simulink library "LU_TEG"  (R2015a)
settings: Solver=ode45  StartTime=0.0  StopTime=10.0  RelTol=1e-3
undefined symbols (not defined in the file): a, a_hxr, B, b_hxr, C_ap, C_cxr, C_hxr, ca1, ca2, ca3, cb1, cb2, cb3, ct1, ct2, Di_cxr, f, k_gap, l, l_cw, l_hxr, l_TEM, M, M_ap, M_cxr, M_hxr, n, N, Nf_hxr, P, plate_fin_hxr_A, side, T1, T1_T2, T_cint, T_hint, tf_hxr, Tune_er, Tune_tr
(part 2 of 2)

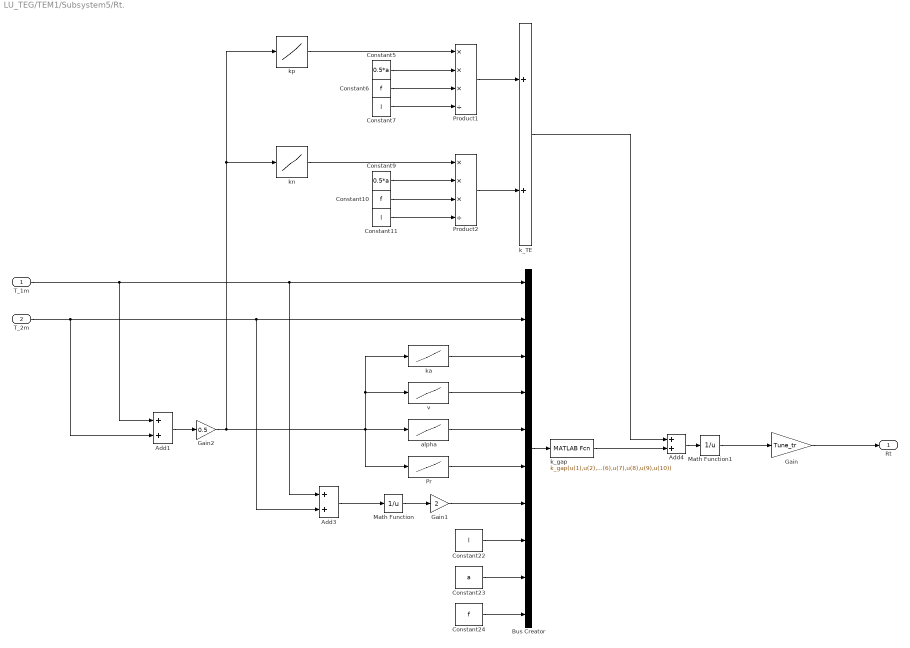
== system LU_TEG/TEM1/Subsystem5/Rt. ==
  T_1m : Inport
  T_2m : Inport  Port=2
  Add1 : Sum
  Add3 : Sum
  Add4 : Sum
  Bus Creator : BusCreator  Inputs=10
  Constant10 : Constant  Value=f
  Constant11 : Constant  Value=l
  Constant22 : Constant  Value=l
  Constant23 : Constant  Value=a
  Constant24 : Constant  Value=f
  Constant5 : Constant  Value=0.5*a
  Constant6 : Constant  Value=f
  Constant7 : Constant  Value=l
  Constant9 : Constant  Value=0.5*a
  Gain : Gain  Gain=Tune_tr
  Gain1 : Gain  Gain=2
  Gain2 : Gain  Gain=0.5
  Math Function : Math  Operator=reciprocal  SaturateOnIntegerOverflow=on
  Math Function1 : Math  Operator=reciprocal  SaturateOnIntegerOverflow=on
  Pr : Lookup_n-D  NumberOfTableDimensions=1  BreakpointsForDimension1=|  Table=|  InterpMethod=Cubic spline  ExtrapMethod=Cubic spline  RndMeth=Simplest  InputSameDT=on
      BreakpointsForDimension1=|
      | [293
      | 313
      | 333
      | 353
      | 373
      | 393
      | 413
      | 433
      | 453
      | 473
      | 493
      | 513
      | 533
      | 553
      | 573
      | 593
      | 613
      | 633
      | 653
      | 673
      | 693
      | 713
      | 733
      | 753
      | 773
      | 793
      | 813
      | 833
      | 853
      | 873
      | 900
      | 920
      | 940
      | 960
      | 980
      | 1000
      | 1020
      | 1040
      | 1060
      | 1080
      | 1100
      | 1120
      | 1140
      | 1160
      | 1180
      | 1200
      | 1220
      | 1240
      | 1260
      | 1280
      | 1300
      | 1320
      | 1340
      | 1360
      | 1380
      | 1400
      | 1420
      | 1440
      | 1460
      | 1480]
      Table=|
      | [0.70868
      | 0.70388
      | 0.69972
      | 0.6964
      | 0.6924
      | 0.68912
      | 0.68696
      | 0.68536
      | 0.68376
      | 0.68216
      | 0.68056
      | 0.68
      | 0.68
      | 0.68
      | 0.68
      | 0.68
      | 0.68052
      | 0.68132
      | 0.68212
      | 0.68292
      | 0.68372
      | 0.68478
      | 0.68598
      | 0.68718
      | 0.68838
      | 0.68958
      | 0.69078
      | 0.69198
      | 0.69318
      | 0.69438
      | 0.696
      | 0.6972
      | 0.6984
      | 0.6996
      | 0.7008
      | 0.702
      | 0.7028
      | 0.7036
      | 0.7046
      | 0.7058
      | 0.707
      | 0.7078
      | 0.7086
      | 0.7094
      | 0.7102
      | 0.711
      | 0.7118
      | 0.7126
      | 0.7134
      | 0.7142
      | 0.715
      | 0.7158
      | 0.7166
      | 0.7174
      | 0.7182
      | 0.719
      | 0.7196
      | 0.7202
      | 0.7208
      | 0.7214
      | ]
  Product1 : Product  Inputs=***/
  Product2 : Product  Inputs=***/
  alpha : Lookup_n-D  NumberOfTableDimensions=1  BreakpointsForDimension1=|  Table=|  InterpMethod=Cubic spline  ExtrapMethod=Cubic spline  RndMeth=Simplest  InputSameDT=on
      BreakpointsForDimension1=|
      | [293
      | 313
      | 333
      | 353
      | 373
      | 393
      | 413
      | 433
      | 453
      | 473
      | 493
      | 513
      | 533
      | 553
      | 573
      | 593
      | 613
      | 633
      | 653
      | 673
      | 693
      | 713
      | 733
      | 753
      | 773
      | 793
      | 813
      | 833
      | 853
      | 873
      | 900
      | 920
      | 940
      | 960
      | 980
      | 1000
      | 1020
      | 1040
      | 1060
      | 1080
      | 1100
      | 1120
      | 1140
      | 1160
      | 1180
      | 1200
      | 1220
      | 1240
      | 1260
      | 1280
      | 1300
      | 1320
      | 1340
      | 1360
      | 1380
      | 1400
      | 1420
      | 1440
      | 1460
      | 1480]
      Table=|
      | [2.14551E-05
      | 2.42197E-05
      | 2.71451E-05
      | 3.01755E-05
      | 3.32992E-05
      | 3.65423E-05
      | 3.98418E-05
      | 4.32631E-05
      | 4.67259E-05
      | 5.03421E-05
      | 5.40342E-05
      | 5.77836E-05
      | 6.16602E-05
      | 6.5511E-05
      | 6.94474E-05
      | 7.35134E-05
      | 7.75786E-05
      | 8.18073E-05
      | 8.60163E-05
      | 9.03078E-05
      | 9.47366E-05
      | 9.91488E-05
      | 0.000103728
      | 0.000108175
      | 0.000112784
      | 0.000117529
      | 0.000122257
      | 0.000127153
      | 0.000132003
      | 0.000137003
      | 0.000142748
      | 0.000147552
      | 0.000152555
      | 0.00015755
      | 0.00016252
      | 0.000167688
      | 0.000172675
      | 0.000178002
      | 0.000183174
      | 0.000188489
      | 0.00019383
      | 0.000199144
      | 0.000204639
      | 0.000210134
      | 0.000215613
      | 0.000221274
      | 0.000226733
      | 0.000232362
      | 0.000238009
      | 0.000243871
      | 0.000249704
      | 0.000255298
      | 0.000261271
      | 0.000267061
      | 0.000273104
      | 0.00027932
      | 0.000285171
      | 0.000290933
      | 0.000297092
      | 0.000303417
      | ]
  k_TE : Sum
  k_gap : MATLABFcn  MATLABFcn=k_gap(u(1),u(2),u(3),u(4),u(5),u(6),u(7),u(8),u(9),u(10))
  ka : Lookup_n-D  NumberOfTableDimensions=1  BreakpointsForDimension1=|  Table=|  InterpMethod=Cubic spline  ExtrapMethod=Cubic spline  RndMeth=Simplest  InputSameDT=on
      BreakpointsForDimension1=|
      | [293
      | 313
      | 333
      | 353
      | 373
      | 393
      | 413
      | 433
      | 453
      | 473
      | 493
      | 513
      | 533
      | 553
      | 573
      | 593
      | 613
      | 633
      | 653
      | 673
      | 693
      | 713
      | 733
      | 753
      | 773
      | 793
      | 813
      | 833
      | 853
      | 873
      | 900
      | 920
      | 940
      | 960
      | 980
      | 1000
      | 1020
      | 1040
      | 1060
      | 1080
      | 1100
      | 1120
      | 1140
      | 1160
      | 1180
      | 1200
      | 1220
      | 1240
      | 1260
      | 1280
      | 1300
      | 1320
      | 1340
      | 1360
      | 1380
      | 1400
      | 1420
      | 1440
      | 1460
      | 1480]
      Table=|
      | [0.02568
      | 0.02716
      | 0.02861
      | 0.03003
      | 0.03142
      | 0.03279
      | 0.03412
      | 0.03544
      | 0.03673
      | 0.03801
      | 0.03926
      | 0.0405
      | 0.04172
      | 0.04293
      | 0.04413
      | 0.04531
      | 0.04648
      | 0.04764
      | 0.04879
      | 0.04993
      | 0.05106
      | 0.05218
      | 0.0533
      | 0.05441
      | 0.05551
      | 0.0566
      | 0.05769
      | 0.05877
      | 0.05985
      | 0.06092
      | 0.06276
      | 0.063736
      | 0.064712
      | 0.065668
      | 0.066604
      | 0.06754
      | 0.068464
      | 0.069388
      | 0.070298
      | 0.071194
      | 0.07209
      | 0.072962
      | 0.073834
      | 0.074696
      | 0.075548
      | 0.0764
      | 0.077236
      | 0.078072
      | 0.0789
      | 0.07972
      | 0.08054
      | 0.081336
      | 0.082132
      | 0.082924
      | 0.083712
      | 0.0845
      | 0.085262
      | 0.086024
      | 0.086786
      | 0.087548]
  kn : Lookup_n-D  NumberOfTableDimensions=1  BreakpointsForDimension1=N(:,1)  Table=N(:,4)  InterpMethod=Cubic spline  ExtrapMethod=Cubic spline  InternalRulePriority=Speed  RndMeth=Simplest  InputSameDT=on
  kp : Lookup_n-D  NumberOfTableDimensions=1  BreakpointsForDimension1=P(:,1)  Table=P(:,4)  InterpMethod=Cubic spline  ExtrapMethod=Cubic spline  InternalRulePriority=Speed  RndMeth=Simplest  InputSameDT=on
  v : Lookup_n-D  NumberOfTableDimensions=1  BreakpointsForDimension1=|  Table=|  InterpMethod=Cubic spline  ExtrapMethod=Cubic spline  RndMeth=Simplest  InputSameDT=on
      BreakpointsForDimension1=|
      | [293
      | 313
      | 333
      | 353
      | 373
      | 393
      | 413
      | 433
      | 453
      | 473
      | 493
      | 513
      | 533
      | 553
      | 573
      | 593
      | 613
      | 633
      | 653
      | 673
      | 693
      | 713
      | 733
      | 753
      | 773
      | 793
      | 813
      | 833
      | 853
      | 873
      | 900
      | 920
      | 940
      | 960
      | 980
      | 1000
      | 1020
      | 1040
      | 1060
      | 1080
      | 1100
      | 1120
      | 1140
      | 1160
      | 1180
      | 1200
      | 1220
      | 1240
      | 1260
      | 1280
      | 1300
      | 1320
      | 1340
      | 1360
      | 1380
      | 1400
      | 1420
      | 1440
      | 1460
      | 1480]
      Table=|
      | [1.50500000000000e-05
      | 1.69228000000000e-05
      | 1.88668000000000e-05
      | 2.08732000000000e-05
      | 2.29612000000000e-05
      | 2.51428000000000e-05
      | 2.74102000000000e-05
      | 2.97182000000000e-05
      | 3.20484000000000e-05
      | 3.45044000000000e-05
      | 3.69604000000000e-05
      | 3.95282000000000e-05
      | 4.21562000000000e-05
      | 4.48034000000000e-05
      | 4.75594000000000e-05
      | 5.03154000000000e-05
      | 5.31650000000000e-05
      | 5.60650000000000e-05
      | 5.89824000000000e-05
      | 6.19984000000000e-05
      | 6.50144000000000e-05
      | 6.81292000000000e-05
      | 7.12972000000000e-05
      | 7.44790000000000e-05
      | 7.77390000000000e-05
      | 8.09990000000000e-05
      | 8.43422000000000e-05
      | 8.77302000000000e-05
      | 9.11350000000000e-05
      | 9.46350000000000e-05
      | 9.93600000000000e-05
      | 0.000102936000000000
      | 0.000106512000000000
      | 0.000110160000000000
      | 0.000113880000000000
      | 0.000117600000000000
      | 0.000121440000000000
      | 0.000125280000000000
      | 0.000129160000000000
      | 0.000133080000000000
      | 0.000137000000000000
      | 0.000141000000000000
      | 0.000145000000000000
      | 0.000149060000000000
      | 0.000153180000000000
      | 0.000157300000000000
      | 0.000161460000000000
      | 0.000165620000000000
      | 0.000169860000000000
      | 0.000174180000000000
      | 0.000178500000000000
      | 0.000182860000000000
      | 0.000187220000000000
      | 0.000191640000000000
      | 0.000196120000000000
      | 0.000200600000000000
      | 0.000205200000000000
      | 0.000209800000000000
      | 0.000214400000000000
      | 0.000219000000000000]
  Rt : Outport
  wires:
  k_TE/1 -> Add4/1
  T_2m/1 -> Add3/2, Bus Creator/2, Add1/2
  Gain2/1 -> alpha/1, ka/1, v/1, Pr/1, kn/1, kp/1
  Add1/1 -> Gain2/1
  Math Function1/1 -> Gain/1
  Add4/1 -> Math Function1/1
  Gain1/1 -> Bus Creator/7
  Constant10/1 -> Product2/3
  Math Function/1 -> Gain1/1
  Constant23/1 -> Bus Creator/9
  Pr/1 -> Bus Creator/6
  Constant24/1 -> Bus Creator/10
  Constant7/1 -> Product1/4
  v/1 -> Bus Creator/4
  Constant11/1 -> Product2/4
  alpha/1 -> Bus Creator/5
  Constant9/1 -> Product2/2
  ka/1 -> Bus Creator/3
  Product2/1 -> k_TE/2
  Constant6/1 -> Product1/3
  Constant5/1 -> Product1/2
  kn/1 -> Product2/1
  kp/1 -> Product1/1
  Constant22/1 -> Bus Creator/8
  Product1/1 -> k_TE/1
  k_gap/1 -> Add4/2
  Bus Creator/1 -> k_gap/1
  T_1m/1 -> Add3/1, Bus Creator/1, Add1/1
  Add3/1 -> Math Function/1
  Gain/1 -> Rt/1

== system LU_TEG/TEMs_CV/Q_TEMs/Q_TEMs. ==
  T_ht : Inport
  T_ct : Inport  Port=2
  Add1 : Sum
  Add2 : Sum  Inputs=+-
  Constant : Constant  Value=l_TEM
  Constant1 : Constant  Value=B-M*a
  Divide : Product  Inputs=**
  Divide1 : Product  Inputs=**/
  Gain : Gain  Gain=0.5
  Insulation : Lookup_n-D  NumberOfTableDimensions=1  BreakpointsForDimension1=|  Table=|  InterpMethod=Cubic spline  ExtrapMethod=Cubic spline  RndMeth=Simplest  InputSameDT=on
      BreakpointsForDimension1=|
      | [273
      | 373
      | 473
      | 573
      | 673
      | 773
      | 873]
      Table=|
      | [0.02
      | 0.023
      | 0.028
      | 0.035
      | 0.046
      | 0.064
      | 0.089]
  Q_ins : Outport
  wires:
  T_ct/1 -> Add2/2, Add1/2
  Gain/1 -> Insulation/1
  Add1/1 -> Gain/1
  T_ht/1 -> Add2/1, Add1/1
  Add2/1 -> Divide/1
  Constant/1 -> Divide1/3
  Divide1/1 -> Divide/2
  Constant1/1 -> Divide1/1
  Divide/1 -> Q_ins/1
  Insulation/1 -> Divide1/2

== system LU_TEG/TEMs_CV/Subsystem4/Subsystem3 ==
  T_exh : Inport
  m_exh : Inport  Port=2
  Bus Creator : BusCreator  Inputs=5
  Constant : Constant  Value=ca1
  Constant1 : Constant  Value=ca2
  Constant2 : Constant  Value=ca3
  Divide4 : Product  Inputs=**/
  Nu : Fcn  Expr=u(1)*u(5)^u(2)*u(4)^u(3)
  Pr : Lookup_n-D  NumberOfTableDimensions=1  BreakpointsForDimension1=|  Table=|  InterpMethod=Cubic spline  ExtrapMethod=Cubic spline  RndMeth=Simplest  InputSameDT=on
      BreakpointsForDimension1=|
      | [293
      | 313
      | 333
      | 353
      | 373
      | 393
      | 413
      | 433
      | 453
      | 473
      | 493
      | 513
      | 533
      | 553
      | 573
      | 593
      | 613
      | 633
      | 653
      | 673
      | 693
      | 713
      | 733
      | 753
      | 773
      | 793
      | 813
      | 833
      | 853
      | 873
      | 900
      | 920
      | 940
      | 960
      | 980
      | 1000
      | 1020
      | 1040
      | 1060
      | 1080
      | 1100
      | 1120
      | 1140
      | 1160
      | 1180
      | 1200
      | 1220
      | 1240
      | 1260
      | 1280
      | 1300
      | 1320
      | 1340
      | 1360
      | 1380
      | 1400
      | 1420
      | 1440
      | 1460
      | 1480]
      Table=|
      | [0.70868
      | 0.70388
      | 0.69972
      | 0.6964
      | 0.6924
      | 0.68912
      | 0.68696
      | 0.68536
      | 0.68376
      | 0.68216
      | 0.68056
      | 0.68
      | 0.68
      | 0.68
      | 0.68
      | 0.68
      | 0.68052
      | 0.68132
      | 0.68212
      | 0.68292
      | 0.68372
      | 0.68478
      | 0.68598
      | 0.68718
      | 0.68838
      | 0.68958
      | 0.69078
      | 0.69198
      | 0.69318
      | 0.69438
      | 0.696
      | 0.6972
      | 0.6984
      | 0.6996
      | 0.7008
      | 0.702
      | 0.7028
      | 0.7036
      | 0.7046
      | 0.7058
      | 0.707
      | 0.7078
      | 0.7086
      | 0.7094
      | 0.7102
      | 0.711
      | 0.7118
      | 0.7126
      | 0.7134
      | 0.7142
      | 0.715
      | 0.7158
      | 0.7166
      | 0.7174
      | 0.7182
      | 0.719
      | 0.7196
      | 0.7202
      | 0.7208
      | 0.7214
      | ]
  Re : Subsystem
  k_exh : Lookup_n-D  NumberOfTableDimensions=1  BreakpointsForDimension1=|  Table=|  InterpMethod=Cubic spline  ExtrapMethod=Cubic spline  RndMeth=Simplest  InputSameDT=on
      BreakpointsForDimension1=|
      | [293
      | 313
      | 333
      | 353
      | 373
      | 393
      | 413
      | 433
      | 453
      | 473
      | 493
      | 513
      | 533
      | 553
      | 573
      | 593
      | 613
      | 633
      | 653
      | 673
      | 693
      | 713
      | 733
      | 753
      | 773
      | 793
      | 813
      | 833
      | 853
      | 873
      | 900
      | 920
      | 940
      | 960
      | 980
      | 1000
      | 1020
      | 1040
      | 1060
      | 1080
      | 1100
      | 1120
      | 1140
      | 1160
      | 1180
      | 1200
      | 1220
      | 1240
      | 1260
      | 1280
      | 1300
      | 1320
      | 1340
      | 1360
      | 1380
      | 1400
      | 1420
      | 1440
      | 1460
      | 1480]
      Table=|
      | [0.02568
      | 0.02716
      | 0.02861
      | 0.03003
      | 0.03142
      | 0.03279
      | 0.03412
      | 0.03544
      | 0.03673
      | 0.03801
      | 0.03926
      | 0.0405
      | 0.04172
      | 0.04293
      | 0.04413
      | 0.04531
      | 0.04648
      | 0.04764
      | 0.04879
      | 0.04993
      | 0.05106
      | 0.05218
      | 0.0533
      | 0.05441
      | 0.05551
      | 0.0566
      | 0.05769
      | 0.05877
      | 0.05985
      | 0.06092
      | 0.06276
      | 0.063736
      | 0.064712
      | 0.065668
      | 0.066604
      | 0.06754
      | 0.068464
      | 0.069388
      | 0.070298
      | 0.071194
      | 0.07209
      | 0.072962
      | 0.073834
      | 0.074696
      | 0.075548
      | 0.0764
      | 0.077236
      | 0.078072
      | 0.0789
      | 0.07972
      | 0.08054
      | 0.081336
      | 0.082132
      | 0.082924
      | 0.083712
      | 0.0845
      | 0.085262
      | 0.086024
      | 0.086786
      | 0.087548]
  h_exh : Outport
  wires:
  Re/1(Re) -> Bus Creator/5
  Pr/1 -> Bus Creator/4
  Re/2(Dh) -> Divide4/3
  k_exh/1 -> Divide4/1
  Divide4/1 -> h_exh/1
  T_exh/1 -> Re/1(T_exh), k_exh/1, Pr/1
  m_exh/1 -> Re/2(m_exh)
  Nu/1 -> Divide4/2
  Constant2/1 -> Bus Creator/3
  Constant1/1 -> Bus Creator/2
  Constant/1 -> Bus Creator/1
  Bus Creator/1 -> Nu/1

== system LU_TEG/TEMs_CV/Subsystem5/Subsystem3 ==
  T_col : Inport
  m_col : Inport  Port=2
  Bus Creator : BusCreator  Inputs=5
  Constant : Constant  Value=cb1
  Constant1 : Constant  Value=cb2
  Constant2 : Constant  Value=Di_cxr
  Constant3 : Constant  Value=cb3
  Divide4 : Product  Inputs=**/
  Nu : Fcn  Expr=u(1)*u(5)^u(2)*u(4)^u(3)
  Pr_col : Lookup_n-D  NumberOfTableDimensions=1  BreakpointsForDimension1=|  Table=|  InterpMethod=Cubic spline  ExtrapMethod=Cubic spline  RndMeth=Simplest  InputSameDT=on
      BreakpointsForDimension1=|
      | [283
      | 293
      | 303
      | 313
      | 323
      | 333
      | 343
      | 353
      | 363
      | 373]
      Table=|
      | [9.47
      | 7.01
      | 5.43
      | 4.34
      | 3.56
      | 2.99
      | 2.56
      | 2.23
      | 1.96
      | 1.75]
  Re : Subsystem
  k_col : Lookup_n-D  NumberOfTableDimensions=1  BreakpointsForDimension1=|  Table=|  InterpMethod=Cubic spline  ExtrapMethod=Cubic spline  RndMeth=Simplest  InputSameDT=on
      BreakpointsForDimension1=|
      | [283
      | 293
      | 303
      | 313
      | 323
      | 333
      | 343
      | 353
      | 363
      | 373]
      Table=|
      | [0.58
      | 0.5984
      | 0.6154
      | 0.63
      | 0.6435
      | 0.6543
      | 0.6631
      | 0.67
      | 0.6753
      | 0.6791]
  h_col : Outport
  wires:
  k_col/1 -> Divide4/1
  Constant2/1 -> Divide4/3
  Re/1(Re) -> Bus Creator/5
  Pr_col/1 -> Bus Creator/4
  m_col/1 -> Re/2(m_col)
  T_col/1 -> Re/1(T_col), k_col/1, Pr_col/1
  Divide4/1 -> h_col/1
  Constant3/1 -> Bus Creator/3
  Constant1/1 -> Bus Creator/2
  Constant/1 -> Bus Creator/1
  Bus Creator/1 -> Nu/1
  Nu/1 -> Divide4/2

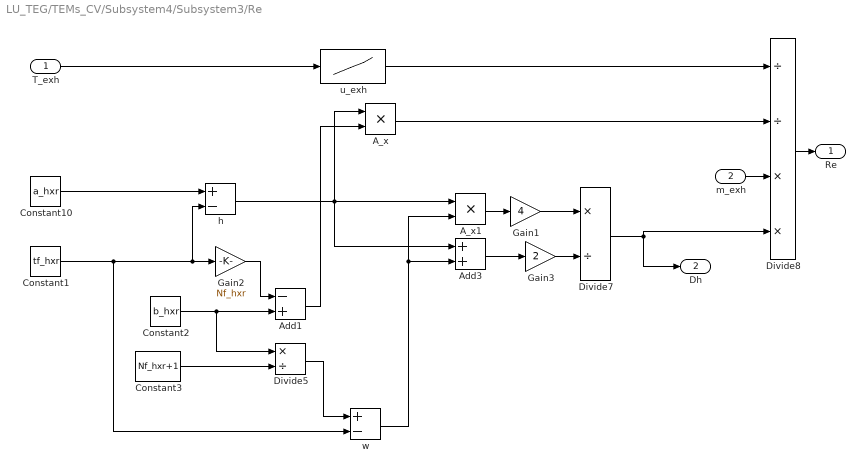
== system LU_TEG/TEMs_CV/Subsystem4/Subsystem3/Re ==
  T_exh : Inport
  m_exh : Inport  Port=2
  A_x : Product  Inputs=**
  A_x1 : Product  Inputs=**
  Add1 : Sum  Inputs=-+
  Add3 : Sum
  Constant1 : Constant  Value=tf_hxr
  Constant10 : Constant  Value=a_hxr
  Constant2 : Constant  Value=b_hxr
  Constant3 : Constant  Value=Nf_hxr+1
  Divide5 : Product  Inputs=*/
  Divide7 : Product  Inputs=*/
  Divide8 : Product  Inputs=//**
  Gain1 : Gain  Gain=4
  Gain2 : Gain  Gain=Nf_hxr
  Gain3 : Gain  Gain=2
  h : Sum  Inputs=+-
  u_exh : Lookup_n-D  NumberOfTableDimensions=1  BreakpointsForDimension1=|  Table=|  InterpMethod=Cubic spline  ExtrapMethod=Cubic spline  RndMeth=Simplest  InputSameDT=on
      BreakpointsForDimension1=|
      | [293
      | 313
      | 333
      | 353
      | 373
      | 393
      | 413
      | 433
      | 453
      | 473
      | 493
      | 513
      | 533
      | 553
      | 573
      | 593
      | 613
      | 633
      | 653
      | 673
      | 693
      | 713
      | 733
      | 753
      | 773
      | 793
      | 813
      | 833
      | 853
      | 873
      | 900
      | 920
      | 940
      | 960
      | 980
      | 1000
      | 1020
      | 1040
      | 1060
      | 1080
      | 1100
      | 1120
      | 1140
      | 1160
      | 1180
      | 1200
      | 1220
      | 1240
      | 1260
      | 1280
      | 1300
      | 1320
      | 1340
      | 1360
      | 1380
      | 1400
      | 1420
      | 1440
      | 1460
      | 1480
      | ]
      Table=|
      | [1.81E-05
      | 1.91E-05
      | 2.00E-05
      | 2.09E-05
      | 2.17E-05
      | 2.26E-05
      | 2.34E-05
      | 2.42E-05
      | 2.50E-05
      | 2.57E-05
      | 2.64E-05
      | 2.72E-05
      | 2.79E-05
      | 2.86E-05
      | 2.93E-05
      | 2.99E-05
      | 3.06E-05
      | 3.12E-05
      | 3.19E-05
      | 3.25E-05
      | 3.31E-05
      | 3.37E-05
      | 3.43E-05
      | 3.49E-05
      | 3.55E-05
      | 3.60E-05
      | 3.66E-05
      | 3.72E-05
      | 3.77E-05
      | 3.82E-05
      | 3.90E-05
      | 3.95E-05
      | 4.00E-05
      | 4.05E-05
      | 4.10E-05
      | 4.15E-05
      | 4.20E-05
      | 4.25E-05
      | 4.30E-05
      | 4.35E-05
      | 4.40E-05
      | 4.44E-05
      | 4.49E-05
      | 4.53E-05
      | 4.58E-05
      | 4.63E-05
      | 4.67E-05
      | 4.71E-05
      | 4.76E-05
      | 4.80E-05
      | 4.85E-05
      | 4.89E-05
      | 4.93E-05
      | 4.97E-05
      | 5.02E-05
      | 5.06E-05
      | 5.10E-05
      | 5.14E-05
      | 5.18E-05
      | 5.22E-05
      | ]
  w : Sum  Inputs=+-
  Re : Outport
  Dh : Outport  Port=2
  wires:
  A_x1/1 -> Gain1/1
  m_exh/1 -> Divide8/3
  A_x/1 -> Divide8/2
  u_exh/1 -> Divide8/1
  Divide7/1 -> Dh/1, Divide8/4
  Add3/1 -> Gain3/1
  Gain3/1 -> Divide7/2
  Gain1/1 -> Divide7/1
  w/1 -> Add3/2, A_x1/2
  Constant1/1 -> Gain2/1, h/2, w/2
  Divide5/1 -> w/1
  Constant3/1 -> Divide5/2
  Add1/1 -> A_x/2
  Gain2/1 -> Add1/1
  Constant2/1 -> Add1/2, Divide5/1
  h/1 -> A_x/1, A_x1/1, Add3/1
  Constant10/1 -> h/1
  T_exh/1 -> u_exh/1
  Divide8/1 -> Re/1

== system LU_TEG/TEMs_CV/Subsystem5/Subsystem3/Re ==
  T_col : Inport
  m_col : Inport  Port=2
  Constant : Constant  Value=4/pi/Di_cxr
  Divide8 : Product  Inputs=/**
  u_col : Lookup_n-D  NumberOfTableDimensions=1  BreakpointsForDimension1=|  Table=|  InterpMethod=Cubic spline  ExtrapMethod=Cubic spline  RndMeth=Simplest  InputSameDT=on
      BreakpointsForDimension1=|
      | [273
      | 274
      | 275
      | 276
      | 277
      | 278
      | 279
      | 280
      | 281
      | 282
      | 283
      | 284
      | 285
      | 286
      | 287
      | 288
      | 289
      | 290
      | 291
      | 292
      | 293
      | 294
      | 295
      | 296
      | 297
      | 298
      | 299
      | 300
      | 301
      | 302
      | 303
      | 304
      | 305
      | 306
      | 307
      | 308
      | 309
      | 310
      | 311
      | 312
      | 313
      | 314
      | 315
      | 316
      | 317
      | 318
      | 319
      | 320
      | 321
      | 322
      | 323
      | 324
      | 325
      | 326
      | 327
      | 328
      | 329
      | 330
      | 331
      | 332
      | 333
      | 334
      | 335
      | 336
      | 337
      | 338
      | 339
      | 340
      | 341
      | 342
      | 343
      | 344
      | 345
      | 346
      | 347
      | 348
      | 349
      | 350
      | 351
      | 352
      | 353
      | 354
      | 355
      | 356
      | 357
      | 358
      | 359
      | 360
      | 361
      | 362
      | 363
      | 364
      | 365
      | 366
      | 367
      | 368
      | 369
      | 370
      | 371
      | 372
      | 373]
      Table=|
      | [0.001792
      | 0.001731
      | 0.001674
      | 0.00162
      | 0.001569
      | 0.00152
      | 0.001473
      | 0.001429
      | 0.001386
      | 0.001346
      | 0.001308
      | 0.001271
      | 0.001236
      | 0.001202
      | 0.00117
      | 0.001139
      | 0.001109
      | 0.001081
      | 0.001054
      | 0.001028
      | 0.001003
      | 0.000979
      | 0.000955
      | 0.000933
      | 0.000911
      | 0.000891
      | 0.000871
      | 0.000852
      | 0.000833
      | 0.000815
      | 0.000798
      | 0.000781
      | 0.000765
      | 0.000749
      | 0.000734
      | 0.00072
      | 0.000705
      | 0.000692
      | 0.000678
      | 0.000666
      | 0.000653
      | 0.000641
      | 0.000629
      | 0.000618
      | 0.000607
      | 0.000596
      | 0.000586
      | 0.000576
      | 0.000566
      | 0.000556
      | 0.000547
      | 0.000538
      | 0.000529
      | 0.000521
      | 0.000512
      | 0.000504
      | 0.000496
      | 0.000489
      | 0.000481
      | 0.000474
      | 0.000467
      | 0.00046
      | 0.000453
      | 0.000447
      | 0.00044
      | 0.000434
      | 0.000428
      | 0.000422
      | 0.000416
      | 0.00041
      | 0.000404
      | 0.000399
      | 0.000394
      | 0.000388
      | 0.000383
      | 0.000378
      | 0.000373
      | 0.000369
      | 0.000364
      | 0.000359
      | 0.000355
      | 0.000351
      | 0.000346
      | 0.000342
      | 0.000338
      | 0.000334
      | 0.00033
      | 0.000326
      | 0.000322
      | 0.000319
      | 0.000315
      | 0.000311
      | 0.000308
      | 0.000304
      | 0.000301
      | 0.000298
      | 0.000295
      | 0.000291
      | 0.000288
      | 0.000285
      | 0.000282
      | ]
  Re : Outport
  wires:
  u_col/1 -> Divide8/1
  T_col/1 -> u_col/1
  Divide8/1 -> Re/1
  m_col/1 -> Divide8/2
  Constant/1 -> Divide8/3
